simulink model "temperature"  (R2021a)
settings: Solver=VariableStepAuto  StartTime=0.0  StopTime=24  MaxStep=0.01  RelTol=1e-3
settings Model: EnablePacing=on  PacingRate=0.250000  Creator=Work  LastModifiedBy=Work

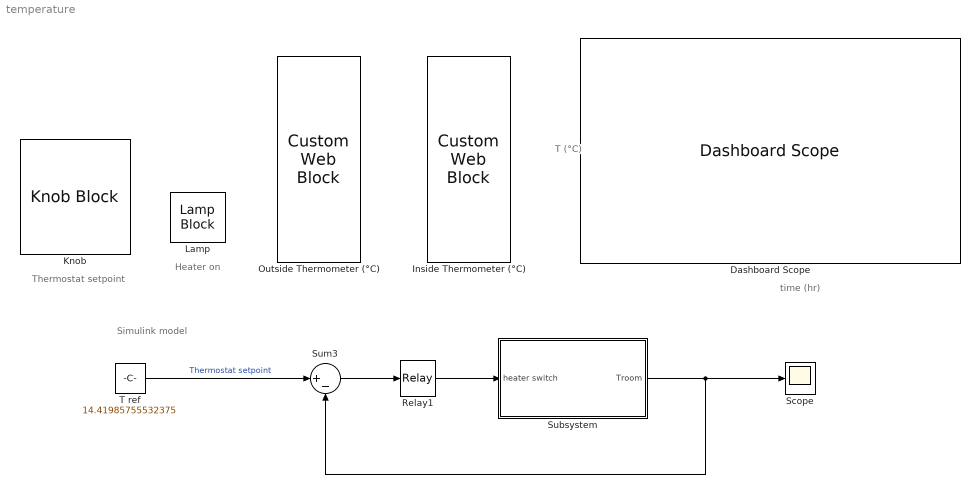
== system temperature ==
  note: Simulink model
  note: time (hr)
  note: Heater on
  note: Thermostat setpoint
  note: T (°C)
  Dashboard Scope : DashboardScope  Ymin=-1  Ymax=51  ScaleAtStop=off
  Inside Thermometer (°C) : CustomWebBlock  LabelPosition=Hide  Configuration="{\"components\":[{\"name\":\"LinearScaleComponent\",\"settings\":{\"bounds\":{\"max\":50,\"min\":0,\"tickInterval\":\"auto\"},\"internalTickHeightScaleFactor\":0.5,\"labelColor\":[38,38,38],\"labelFont\":{\"font\":\"Arial\",\"fontSize\":12},\"labelTransparency\":1,\"needleImage\":{\"size\":[0,0],\"src\":\"\",\"srcOrientation\":\"vertical\"},\"needleOffset\":[0,0],\"needleSize\":{\"height\":0,\"width\":0},\"position\":[0.07305119926199262,0.12572337962962962,0.3736979166666667,0.680984778597786],\"scaleColors\":[],\"scaleColorsSize\":0.2,\"showLabels\":1,\"showMinorTicks\":0,\"showSpanLine\":1,\"showTicks\":1,\"tickColor\":[0,0,0],\"tickTransparency\":1,\"valueBarColor\":[194,0,0],\"valueBarOffset\":0,\"valueBarSize\":0.55,\"valueBarTransparency\":0.8}},{\"name\":\"BackgroundImageComponent\",\"settings\":{\"image\":{\"size\":[154,384],\"src\":\"data:image\\/svg+xml;base64,PHN2ZyB3aWR0aD0iMTU0IiBoZWlnaHQ9IjM4NCIgeG1sbnM9Imh0dHA6Ly93d3cudzMub3JnLzIwMDAvc3ZnIiB4bWxuczp4bGluaz0iaHR0cDovL3d3dy53My5vcmcvMTk5OS94bGluayIgb3ZlcmZsb3c9ImhpZGRlbiI+PGRlZnM+PGNsaXBQYXRoIGlkPSJjbGlwMCI+PHBhdGggZD0iTTAgMCAxNTQgMCAxNTQgMzg0IDAgMzg0WiIgZmlsbC1ydWxlPSJldmVub2RkIiBjbGlwLXJ1bGU9ImV2ZW5vZGQiLz48L2NsaXBQYXRoPjwvZGVmcz48ZyBjbGlwLXBhdGg9InVybCgjY2xpcDApIj48cmVjdCB4PSIwIiB5PSIwIiB3aWR0aD0i ...(+1892 chars)\",\"srcOrientation\":\"vertical\"},\"position\":[0,0,1,1],\"scaleMode\":\"0\"}},{\"name\":\"ForegroundImageComponent\",\"settings\":{\"image\":{\"size\":[0,0],\"src\":\"default\",\"srcOrientation\":[]},\"isForeground\":1,\"position\":[0,0,1,1],\"scaleMode\":\"0\"}}],\"settings\":{\"BindingType\":\"signal\",\"aspectRatio\":0.4010416666666667,\"fixedAspectRatio\":\"on\",\"orientation\":\"vertical\",\"value\":0},\"type\":\"LinearGauge\"}"
  Knob : KnobBlock  ScaleMax=50
  Lamp : LampBlock
  Outside Thermometer (°C) : CustomWebBlock  LabelPosition=Hide  Configuration="{\"components\":[{\"name\":\"LinearScaleComponent\",\"settings\":{\"bounds\":{\"max\":50,\"min\":0,\"tickInterval\":\"auto\"},\"internalTickHeightScaleFactor\":0.5,\"labelColor\":[38,38,38],\"labelFont\":{\"font\":\"Arial\",\"fontSize\":12},\"labelTransparency\":1,\"needleImage\":{\"size\":[0,0],\"src\":\"\",\"srcOrientation\":\"vertical\"},\"needleOffset\":[0,0],\"needleSize\":{\"height\":0,\"width\":0},\"position\":[0.07305119926199262,0.12572337962962962,0.3736979166666667,0.680984778597786],\"scaleColors\":[],\"scaleColorsSize\":0.2,\"showLabels\":1,\"showMinorTicks\":0,\"showSpanLine\":1,\"showTicks\":1,\"tickColor\":[0,0,0],\"tickTransparency\":1,\"valueBarColor\":[194,0,0],\"valueBarOffset\":0,\"valueBarSize\":0.55,\"valueBarTransparency\":0.8}},{\"name\":\"BackgroundImageComponent\",\"settings\":{\"image\":{\"size\":[154,384],\"src\":\"data:image\\/svg+xml;base64,PHN2ZyB3aWR0aD0iMTU0IiBoZWlnaHQ9IjM4NCIgeG1sbnM9Imh0dHA6Ly93d3cudzMub3JnLzIwMDAvc3ZnIiB4bWxuczp4bGluaz0iaHR0cDovL3d3dy53My5vcmcvMTk5OS94bGluayIgb3ZlcmZsb3c9ImhpZGRlbiI+PGRlZnM+PGNsaXBQYXRoIGlkPSJjbGlwMCI+PHBhdGggZD0iTTAgMCAxNTQgMCAxNTQgMzg0IDAgMzg0WiIgZmlsbC1ydWxlPSJldmVub2RkIiBjbGlwLXJ1bGU9ImV2ZW5vZGQiLz48L2NsaXBQYXRoPjwvZGVmcz48ZyBjbGlwLXBhdGg9InVybCgjY2xpcDApIj48cmVjdCB4PSIwIiB5PSIwIiB3aWR0aD0i ...(+1892 chars)\",\"srcOrientation\":\"vertical\"},\"position\":[0,0,1,1],\"scaleMode\":\"0\"}},{\"name\":\"ForegroundImageComponent\",\"settings\":{\"image\":{\"size\":[0,0],\"src\":\"default\",\"srcOrientation\":[]},\"isForeground\":1,\"position\":[0,0,1,1],\"scaleMode\":\"0\"}}],\"settings\":{\"BindingType\":\"signal\",\"aspectRatio\":0.4010416666666667,\"fixedAspectRatio\":\"on\",\"orientation\":\"vertical\",\"value\":0},\"type\":\"LinearGauge\"}"
  Relay1 : Relay  OnSwitchValue=2  OffSwitchValue=-2
  Scope : Scope
  Subsystem : Subsystem
  Sum3 : Sum  Inputs=|+-  InputSameDT=on  SaturateOnIntegerOverflow=on  OutDataTypeStr=Inherit: Same as first input
  T ref : Constant  Value=14.41985755532375  SampleTime=0.01
  wires:
  Sum3/1 -> Relay1/1
  T ref/1 -> Sum3/1  "Thermostat setpoint"
  Subsystem/1(Troom) -> Scope/1, Sum3/2
  Relay1/1 -> Subsystem/1(heater switch)

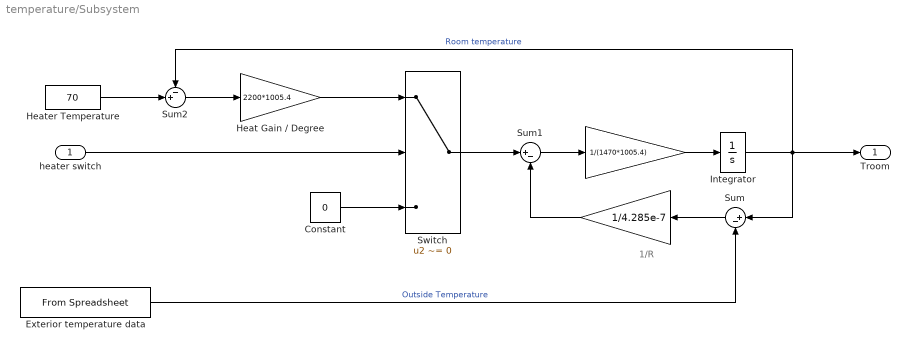
== system temperature/Subsystem ==
  note: 1/R
  heater switch : Inport
  " " : Gain  Gain=1/4.285e-7  SaturateOnIntegerOverflow=on  OutDataTypeStr=Inherit: Same as input  ParamDataTypeStr=Inherit: Same as input
  "  " : Gain  Gain=1/(1470*1005.4)  SaturateOnIntegerOverflow=on  OutDataTypeStr=Inherit: Same as input  ParamDataTypeStr=Inherit: Same as input
  Constant : Constant  Value=0
  Exterior temperature data : FromSpreadsheet  FileName=TData.xlsx
  Heat Gain / Degree : Gain  Gain=2200*1005.4
  Heater Temperature : Constant  Value=70
  Integrator : Integrator  InitialCondition=20
  Sum : Sum  Inputs=|+-
  Sum1 : Sum  Inputs=|+-  InputSameDT=on  SaturateOnIntegerOverflow=on  OutDataTypeStr=Inherit: Same as first input
  Sum2 : Sum  Inputs=-+|
  Switch : Switch  Criteria=u2 ~= 0
  Troom : Outport
  wires:
  Integrator/1 -> Sum/1, Sum2/1, Troom/1  "Room temperature"
  Exterior temperature data/1 -> Sum/2  "Outside Temperature"
  Switch/1 -> Sum1/1
  "  "/1 -> Integrator/1
  Heat Gain / Degree/1 -> Switch/1
  " "/1 -> Sum1/2
  Sum1/1 -> "  "/1
  Heater Temperature/1 -> Sum2/2
  Sum2/1 -> Heat Gain / Degree/1
  Sum/1 -> " "/1
  heater switch/1 -> Switch/2
  Constant/1 -> Switch/3
